simulink model "Encoder_Zynq_V25"  (R2021a)
settings: Solver=FixedStepDiscrete  StartTime=0.0  StopTime=SimulationsDauer  RelTol=1e-3
values from neighbouring files (symbols this model uses):
  f_ISR = 40e3    (= 40000)    [Script_Encoder_Zynq.m]
  IncPerTurn = 1024    [Script_Encoder_Zynq.m]
  inital_zero_speed_timeout = speed_timeout_in_s*f_fpga    (= 10000)    [Script_Encoder_Zynq.m]
  n_max = 6000    [Script_Encoder_Zynq.m]
  OmegaPerOverSampl = 500*((2*pi)/60)    (= 52.3598775598)    [Script_Encoder_Zynq.m]
  Periode = abs(1/Striche_pro_Sekunde)    [Script_Encoder_Zynq.m]
  Phase_Delay_A = Periode/8    [Script_Encoder_Zynq.m]
  Phase_Delay_B = -Periode/8    [Script_Encoder_Zynq.m]
  PolePair = 1    [Script_Encoder_Zynq.m]
  QuadratureFactor = 4    [Script_Encoder_Zynq.m]
  reciprocal_iterations = 3    [Script_Encoder_Zynq.m]
  T_50MHz = 1/f_50MHz    (= 1e-08)    [Script_Encoder_Zynq.m]
  T_mech = 1e-08    [Script_Encoder_Zynq.m]
undefined symbols (not defined in the file or in its folder): DiscIntNeverNeededParam, Newton, Raphson
libraries: hdlsllib x17, dspsrcs4 x3, simulink x2, dspswit3 x2, spsEdgeDetectorLib x2, simulink_extras x1, spspowerguiLib x1
(part 2 of 3)

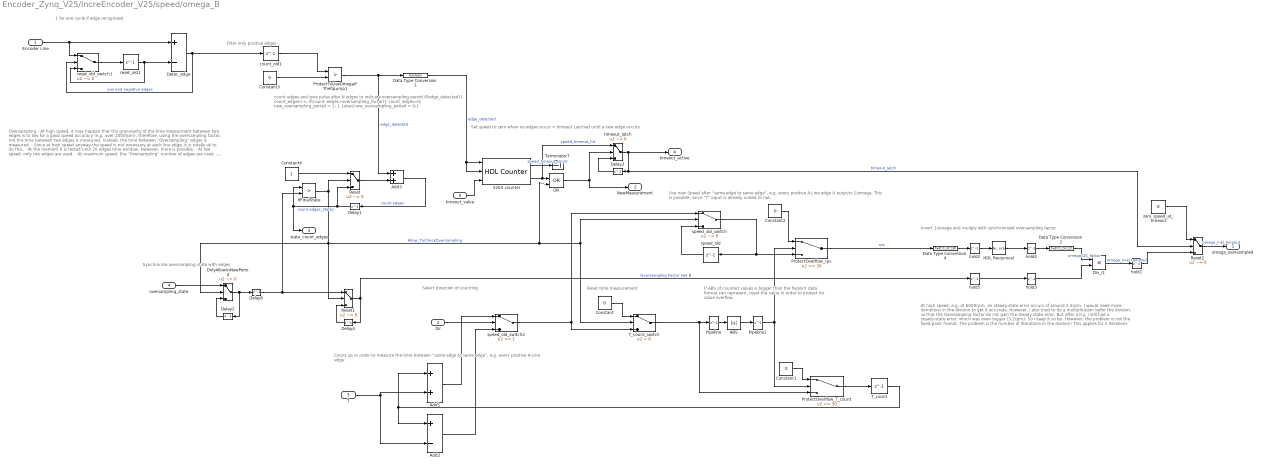
== system Encoder_Zynq_V25/IncreEncoder_V25/speed/omega_B ==
  note: Oversampling
      | - At high speed, it may happen that the granularity of the time measurment between
      | two edges is to low for a good speed accuracy (e.g. over 2000rpm), therefore, using
      | the oversampling factor, not the time between two edges is measured. Instead, the
      | time between "Oversampling" edges is measured.
      | - Since at high speed anyway the speed is not necessary at each line edge,
      |  it is totally ok to do this.
      | - At the moment it is tested until 20 edges time window. However, more is possible.
      | - At low speed, only two edges are used.
      | - At maximum speed, the "Oversampling" number of edges are used.
      | - Between them, a linear factor is used.
      | - Using the OverSampling number also at low speed is not possible,
      |  since the fixpoint range must be quite high! (fixdt(1,36,30) is used at the moment)
  note: Count up in order to measure the time between "same edge to same edge", e.g. every positive A-Line edge
  note: Reset time measurement
  note: 1 for one cycle if edge recognized
  note: Use new Speed after "same edge to same edge", e.g. every positive A-Line edge
      | It outputs 1/omega. This is possible, since "T" input is already scaled to rad.
  note: Select direction of counting
  note: If ABS of counted values is bigger than the
      | fixpoint data format can represent, reset the
      | value in order to protect for value overflow.
  note: Filter only positive edges
  note: count edges and give pulse after N edges to indicate oversampling period
      | if(edge_detected){
      | 	count_edges++;
      | 	if(count_edges>oversampling_factor){
      | 		count_edges=0;
      | 		new_oversampling_period = 1;
      | 	}
      | }else{new_oversampling_period = 0;}
  note: Synchronize oversampling state with edges
  note: At high speed, e.g. at 6000rpm, an steady-state error occurs of around 2.5rpm. I would need more iterrations in the division to get it accurate.
      | However, i also tried to do a multiplication befor the division, so that the Oversampling factor do not gain the steady-state error.
      | But after a try, i still had a steady-state error, which was even bigger (3,2rpm). So i keep it so far.
      | However, the problem is not the fixed-point fromat. The problem is the number of itterations in the division!
      | This applies for 3 iterations
  note: Invert 1/omega and muliply with synchronized oversampling factor
  note: Set speed to zero when no edges occur = timeout
      | Latched until a new edge occurs
  Encoder Line : Inport
  Dir : Inport  Port=2
  T : Inport  Port=3
  oversampling_state : Inport  Port=4
  timeout_value : Inport  Port=5  OutDataTypeStr=uint32
  32bit counter : hdlsllib/Sources/HDL Counter  CountType=Count limited  CountInit=0  CountStep=1  CountMax=inital_zero_speed_timeout  CountFromType=Initial value  CountFrom=0  CountResetPort=on  CountLoadPort=on  CountEnbPort=off  CountDirPort=off  CountHitOutputPort=on  CountDataType=Unsigned  CountWordLen=32  CountFracLen=0  CountSampTime=1
  ABS : Abs
  Add1 : Sum  OutDataTypeStr=Inherit: Same as first input
  Add2 : Sum  Inputs=+-  OutDataTypeStr=Inherit: Same as first input
  Add3 : Sum  OutDataTypeStr=Inherit: Same as accumulator
  Constant : Constant  Value=0  OutDataTypeStr=fixdt(1,38,32)  SampleTime=-1
  Constant1 : Constant  Value=0  OutDataTypeStr=fixdt(1,38,32)  SampleTime=-1
  Constant2 : Constant  Value=0  OutDataTypeStr=fixdt(1,38,32)  SampleTime=-1
  Constant3 : Constant  Value=0  OutDataTypeStr=int8  SampleTime=-1
  Constant4 : Constant  OutDataTypeStr=int8  SampleTime=T_50MHz
  Data Type Conversion1 : DataTypeConversion  OutDataTypeStr=boolean
  Data Type Conversion2 : DataTypeConversion  OutDataTypeStr=fixdt(1,24,12)
  Data Type Conversion4 : DataTypeConversion  OutDataTypeStr=fixdt(1,32,18)
  Delay{1..4,8} (5 alike) : Delay  DelayLength=1  InitialCondition=0
  Detec_edge : Sum  Inputs=+-  AccumDataTypeStr=int8  OutDataTypeStr=int8
  Div_i1 : Product  Inputs=**  OutDataTypeStr=fixdt(1,24,11)  RndMeth=Simplest  SaturateOnIntegerOverflow=on
  HDL Reciprocal : Reciprocal  NumberOfIterations=reciprocal_iterations
  IfFinalState : RelationalOperator  Operator=>  OutDataTypeStr=boolean  RndMeth=Nearest
  OR : Logic  Operator=OR  IconShape=distinctive  AllPortsSameDT=off  OutDataTypeStr=boolean
  OnlyAllowInNewPeriod : Switch  Criteria=u2 ~= 0  Threshold=0.5  OutDataTypeStr=fixdt(0,16,0)
  Pipeline : Delay  DelayLength=1
  Pipeline1 : Delay  DelayLength=1
  ProtectOverflow_T_count : Switch  Threshold=30
  ProtectOverflow_rps : Switch  Threshold=30  OutDataTypeStr=fixdt(1,38,32)
  ProtectToUseOmegaIfThetaJump1 : RelationalOperator  Operator=>  OutDataTypeStr=fixdt(1,16)  RndMeth=Nearest
  Reset : Switch  Criteria=u2 ~= 0  Threshold=0.5  OutDataTypeStr=fixdt(1,24,11)
  Reset1 : Switch  Criteria=u2 ~= 0  Threshold=0.5  OutDataTypeStr=Inherit: Inherit via back propagation
  Reset2 : Switch  Criteria=u2 ~= 0  Threshold=0.5  OutDataTypeStr=Inherit: Inherit via back propagation
  T_count : Delay  DelayLength=1
  T_count_switch : Switch  Criteria=u2 > Threshold
  Terminator7 : Terminator
  count_old1 : Delay  DelayLength=1
  hold1 : Delay
  hold{2..5} (4 alike) : Delay  DelayLength=1
  reset_old1 : Delay  DelayLength=1
  reset_old_switch1 : Switch  Criteria=u2 ~= 0
  speed_old : Delay  DelayLength=1
  speed_old_switch : Switch  Criteria=u2 ~= 0  OutDataTypeStr=fixdt(1,38,32)
  speed_old_switch2 : Switch  Threshold=1
  timeout_latch : Switch  Criteria=u2 ~= 0  Threshold=0.5  OutDataTypeStr=Inherit: Inherit via back propagation
  zero_speed_at_timeout : Constant  Value=0  OutDataTypeStr=fixdt(1,24,12)  SampleTime=-1
  omega_oversampled : Outport  VectorParamsAs1DForOutWhenUnconnected=off
  NewMeasurement : Outport  Port=2  VectorParamsAs1DForOutWhenUnconnected=off
  state_count_edges : Outport  Port=3  VectorParamsAs1DForOutWhenUnconnected=off
  timeout_active : Outport  Port=4  OutDataTypeStr=boolean  VectorParamsAs1DForOutWhenUnconnected=off
  wires:
  Constant/1 -> T_count_switch/1
  Constant1/1 -> ProtectOverflow_T_count/1
  Constant2/1 -> ProtectOverflow_rps/1
  speed_old_switch/1 -> ProtectOverflow_rps/3, speed_old/1
  speed_old/1 -> speed_old_switch/3
  T/1 -> Add1/2, Add2/2
  ProtectOverflow_T_count/1 -> T_count/1
  T_count/1 -> Add2/1, Add1/1
  speed_old_switch2/1 -> speed_old_switch/1, T_count_switch/3
  count_old1/1 -> ProtectToUseOmegaIfThetaJump1/1
  Constant3/1 -> ProtectToUseOmegaIfThetaJump1/2
  Encoder Line/1 -> reset_old_switch1/1, Detec_edge/1
  reset_old_switch1/1 -> reset_old1/1
  reset_old1/1 -> reset_old_switch1/3, Detec_edge/2
  Detec_edge/1 -> reset_old_switch1/2, count_old1/1  "pos and negative edges"
  Dir/1 -> speed_old_switch2/2
  Add1/1 -> speed_old_switch2/1
  Add2/1 -> speed_old_switch2/3
  T_count_switch/1 -> Pipeline/1, ProtectOverflow_T_count/3
  ABS/1 -> Pipeline1/1
  Pipeline/1 -> ABS/1
  Pipeline1/1 -> ProtectOverflow_T_count/2, ProtectOverflow_rps/2
  IfFinalState/1 -> OR/2, speed_old_switch/2, T_count_switch/2, Reset1/2, OnlyAllowInNewPeriod/2, Reset/2  "Allow_ToCheckOversampling"
  OnlyAllowInNewPeriod/1 -> Delay2/1, Delay8/1
  Delay1/1 -> Reset/3, state_count_edges/1, IfFinalState/1  "count edges_states"
  Add3/1 -> Delay1/1  "count edges"
  Reset/1 -> Add3/2
  Constant4/1 -> Reset/1
  Reset1/1 -> Delay4/1, hold5/1  "Oversampling Factor Not B"
  Delay2/1 -> OnlyAllowInNewPeriod/3
  oversampling_state/1 -> OnlyAllowInNewPeriod/1
  Delay4/1 -> Reset1/3
  Delay8/1 -> Reset1/1, IfFinalState/2
  ProtectToUseOmegaIfThetaJump1/1 -> Add3/1, Data Type Conversion1/1  "edge_detected"
  32bit counter/2 -> OR/1, timeout_latch/1  "speed_timeout_hit"
  OR/1 -> NewMeasurement/1, timeout_latch/2
  Div_i1/1 -> hold1/1  "omega_oversampled"
  hold2/1 -> HDL Reciprocal/1
  hold4/1 -> Data Type Conversion2/1
  HDL Reciprocal/1 -> hold4/1
  hold5/1 -> hold3/1
  hold3/1 -> Div_i1/2
  Data Type Conversion2/1 -> Div_i1/1  "omega/OS_factor"
  ProtectOverflow_rps/1 -> Data Type Conversion4/1  "rps"
  Data Type Conversion4/1 -> hold2/1
  zero_speed_at_timeout/1 -> Reset2/1
  Reset2/1 -> omega_oversampled/1  "omega_inkl_timeout"
  timeout_latch/1 -> timeout_active/1, Reset2/2, Delay3/1  "timeout_latch"
  Delay3/1 -> timeout_latch/3
  Data Type Conversion1/1 -> 32bit counter/2, 32bit counter/1  "edge_detected"
  timeout_value/1 -> 32bit counter/3
  32bit counter/1 -> Terminator7/1  "speed_timeout_count"
  hold1/1 -> Reset2/3

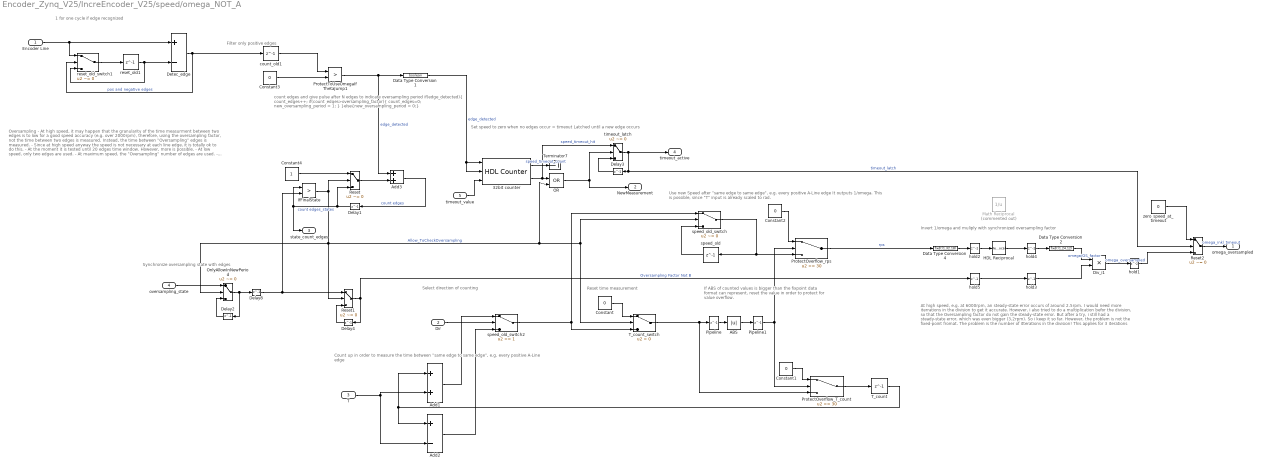
== system Encoder_Zynq_V25/IncreEncoder_V25/speed/omega_NOT_A ==
  note: Oversampling
      | - At high speed, it may happen that the granularity of the time measurment between
      | two edges is to low for a good speed accuracy (e.g. over 2000rpm), therefore, using
      | the oversampling factor, not the time between two edges is measured. Instead, the
      | time between "Oversampling" edges is measured.
      | - Since at high speed anyway the speed is not necessary at each line edge,
      |  it is totally ok to do this.
      | - At the moment it is tested until 20 edges time window. However, more is possible.
      | - At low speed, only two edges are used.
      | - At maximum speed, the "Oversampling" number of edges are used.
      | - Between them, a linear factor is used.
      | - Using the OverSampling number also at low speed is not possible,
      |  since the fixpoint range must be quite high! (fixdt(1,36,30) is used at the moment)
  note: Count up in order to measure the time between "same edge to same edge", e.g. every positive A-Line edge
  note: Reset time measurement
  note: 1 for one cycle if edge recognized
  note: Use new Speed after "same edge to same edge", e.g. every positive A-Line edge
      | It outputs 1/omega. This is possible, since "T" input is already scaled to rad.
  note: Select direction of counting
  note: If ABS of counted values is bigger than the
      | fixpoint data format can represent, reset the
      | value in order to protect for value overflow.
  note: Filter only positive edges
  note: count edges and give pulse after N edges to indicate oversampling period
      | if(edge_detected){
      | 	count_edges++;
      | 	if(count_edges>oversampling_factor){
      | 		count_edges=0;
      | 		new_oversampling_period = 1;
      | 	}
      | }else{new_oversampling_period = 0;}
  note: Synchronize oversampling state with edges
  note: At high speed, e.g. at 6000rpm, an steady-state error occurs of around 2.5rpm. I would need more iterrations in the division to get it accurate.
      | However, i also tried to do a multiplication befor the division, so that the Oversampling factor do not gain the steady-state error.
      | But after a try, i still had a steady-state error, which was even bigger (3,2rpm). So i keep it so far.
      | However, the problem is not the fixed-point fromat. The problem is the number of itterations in the division!
      | This applies for 3 iterations
  note: Invert 1/omega and muliply with synchronized oversampling factor
  note: Set speed to zero when no edges occur = timeout
      | Latched until a new edge occurs
  Encoder Line : Inport
  Dir : Inport  Port=2
  T : Inport  Port=3
  oversampling_state : Inport  Port=4
  timeout_value : Inport  Port=5  OutDataTypeStr=uint32
  32bit counter : hdlsllib/Sources/HDL Counter  CountType=Count limited  CountInit=0  CountStep=1  CountMax=inital_zero_speed_timeout  CountFromType=Initial value  CountFrom=0  CountResetPort=on  CountLoadPort=on  CountEnbPort=off  CountDirPort=off  CountHitOutputPort=on  CountDataType=Unsigned  CountWordLen=32  CountFracLen=0  CountSampTime=1
  ABS : Abs
  Add1 : Sum  OutDataTypeStr=Inherit: Same as first input
  Add2 : Sum  Inputs=+-  OutDataTypeStr=Inherit: Same as first input
  Add3 : Sum  OutDataTypeStr=Inherit: Same as accumulator
  Constant : Constant  Value=0  OutDataTypeStr=fixdt(1,38,32)  SampleTime=-1
  Constant1 : Constant  Value=0  OutDataTypeStr=fixdt(1,38,32)  SampleTime=-1
  Constant2 : Constant  Value=0  OutDataTypeStr=fixdt(1,38,32)  SampleTime=-1
  Constant3 : Constant  Value=0  OutDataTypeStr=int8  SampleTime=-1
  Constant4 : Constant  OutDataTypeStr=int8  SampleTime=T_50MHz
  Data Type Conversion1 : DataTypeConversion  OutDataTypeStr=boolean
  Data Type Conversion2 : DataTypeConversion  OutDataTypeStr=fixdt(1,24,12)
  Data Type Conversion4 : DataTypeConversion  OutDataTypeStr=fixdt(1,32,18)
  Delay{1..4,8} (5 alike) : Delay  DelayLength=1  InitialCondition=0
  Detec_edge : Sum  Inputs=+-  AccumDataTypeStr=int8  OutDataTypeStr=int8
  Div_i1 : Product  Inputs=**  OutDataTypeStr=fixdt(1,24,11)  RndMeth=Simplest  SaturateOnIntegerOverflow=on
  HDL Reciprocal : Reciprocal  NumberOfIterations=reciprocal_iterations
  IfFinalState : RelationalOperator  Operator=>  OutDataTypeStr=boolean  RndMeth=Nearest
  Math Reciprocal : Math  Commented=on  Operator=reciprocal  AlgorithmMethod=Newton-Raphson  SignedPower=on  Iterations=reciprocal_iterations  SaturateOnIntegerOverflow=on
  OR : Logic  Operator=OR  IconShape=distinctive  AllPortsSameDT=off  OutDataTypeStr=boolean
  OnlyAllowInNewPeriod : Switch  Criteria=u2 ~= 0  Threshold=0.5  OutDataTypeStr=fixdt(0,16,0)
  Pipeline : Delay  DelayLength=1
  Pipeline1 : Delay  DelayLength=1
  ProtectOverflow_T_count : Switch  Threshold=30
  ProtectOverflow_rps : Switch  Threshold=30  OutDataTypeStr=fixdt(1,38,32)
  ProtectToUseOmegaIfThetaJump1 : RelationalOperator  Operator=>  OutDataTypeStr=fixdt(1,16)  RndMeth=Nearest
  Reset : Switch  Criteria=u2 ~= 0  Threshold=0.5  OutDataTypeStr=fixdt(1,24,11)
  Reset1 : Switch  Criteria=u2 ~= 0  Threshold=0.5  OutDataTypeStr=Inherit: Inherit via back propagation
  Reset2 : Switch  Criteria=u2 ~= 0  Threshold=0.5  OutDataTypeStr=Inherit: Inherit via back propagation
  T_count : Delay  DelayLength=1
  T_count_switch : Switch  Criteria=u2 > Threshold
  Terminator7 : Terminator
  count_old1 : Delay  DelayLength=1
  hold1 : Delay
  hold{2..5} (4 alike) : Delay  DelayLength=1
  reset_old1 : Delay  DelayLength=1
  reset_old_switch1 : Switch  Criteria=u2 ~= 0
  speed_old : Delay  DelayLength=1
  speed_old_switch : Switch  Criteria=u2 ~= 0  OutDataTypeStr=fixdt(1,38,32)
  speed_old_switch2 : Switch  Threshold=1
  timeout_latch : Switch  Criteria=u2 ~= 0  Threshold=0.5  OutDataTypeStr=Inherit: Inherit via back propagation
  zero_speed_at_timeout : Constant  Value=0  OutDataTypeStr=fixdt(1,24,12)  SampleTime=-1
  omega_oversampled : Outport  VectorParamsAs1DForOutWhenUnconnected=off
  NewMeasurement : Outport  Port=2  VectorParamsAs1DForOutWhenUnconnected=off
  state_count_edges : Outport  Port=3  VectorParamsAs1DForOutWhenUnconnected=off
  timeout_active : Outport  Port=4  OutDataTypeStr=boolean  VectorParamsAs1DForOutWhenUnconnected=off
  wires:
  Constant/1 -> T_count_switch/1
  Constant1/1 -> ProtectOverflow_T_count/1
  Constant2/1 -> ProtectOverflow_rps/1
  speed_old_switch/1 -> ProtectOverflow_rps/3, speed_old/1
  speed_old/1 -> speed_old_switch/3
  T/1 -> Add1/2, Add2/2
  ProtectOverflow_T_count/1 -> T_count/1
  T_count/1 -> Add2/1, Add1/1
  speed_old_switch2/1 -> speed_old_switch/1, T_count_switch/3
  count_old1/1 -> ProtectToUseOmegaIfThetaJump1/1
  Constant3/1 -> ProtectToUseOmegaIfThetaJump1/2
  Encoder Line/1 -> reset_old_switch1/1, Detec_edge/1
  reset_old_switch1/1 -> reset_old1/1
  reset_old1/1 -> reset_old_switch1/3, Detec_edge/2
  Detec_edge/1 -> reset_old_switch1/2, count_old1/1  "pos and negative edges"
  Dir/1 -> speed_old_switch2/2
  Add1/1 -> speed_old_switch2/1
  Add2/1 -> speed_old_switch2/3
  T_count_switch/1 -> Pipeline/1, ProtectOverflow_T_count/3
  ABS/1 -> Pipeline1/1
  Pipeline/1 -> ABS/1
  Pipeline1/1 -> ProtectOverflow_T_count/2, ProtectOverflow_rps/2
  IfFinalState/1 -> OR/2, speed_old_switch/2, T_count_switch/2, Reset1/2, OnlyAllowInNewPeriod/2, Reset/2  "Allow_ToCheckOversampling"
  OnlyAllowInNewPeriod/1 -> Delay2/1, Delay8/1
  Delay1/1 -> Reset/3, state_count_edges/1, IfFinalState/1  "count edges_states"
  Add3/1 -> Delay1/1  "count edges"
  Reset/1 -> Add3/2
  Constant4/1 -> Reset/1
  Reset1/1 -> Delay4/1, hold5/1  "Oversampling Factor Not B"
  Delay2/1 -> OnlyAllowInNewPeriod/3
  oversampling_state/1 -> OnlyAllowInNewPeriod/1
  Delay4/1 -> Reset1/3
  Delay8/1 -> Reset1/1, IfFinalState/2
  ProtectToUseOmegaIfThetaJump1/1 -> Add3/1, Data Type Conversion1/1  "edge_detected"
  32bit counter/2 -> OR/1, timeout_latch/1  "speed_timeout_hit"
  OR/1 -> NewMeasurement/1, timeout_latch/2
  Div_i1/1 -> hold1/1  "omega_oversampled"
  hold2/1 -> HDL Reciprocal/1
  hold4/1 -> Data Type Conversion2/1
  HDL Reciprocal/1 -> hold4/1
  hold5/1 -> hold3/1
  hold3/1 -> Div_i1/2
  Data Type Conversion2/1 -> Div_i1/1  "omega/OS_factor"
  ProtectOverflow_rps/1 -> Data Type Conversion4/1  "rps"
  Data Type Conversion4/1 -> hold2/1
  zero_speed_at_timeout/1 -> Reset2/1
  Reset2/1 -> omega_oversampled/1  "omega_inkl_timeout"
  timeout_latch/1 -> timeout_active/1, Reset2/2, Delay3/1  "timeout_latch"
  Delay3/1 -> timeout_latch/3
  Data Type Conversion1/1 -> 32bit counter/2, 32bit counter/1  "edge_detected"
  timeout_value/1 -> 32bit counter/3
  32bit counter/1 -> Terminator7/1  "speed_timeout_count"
  hold1/1 -> Reset2/3

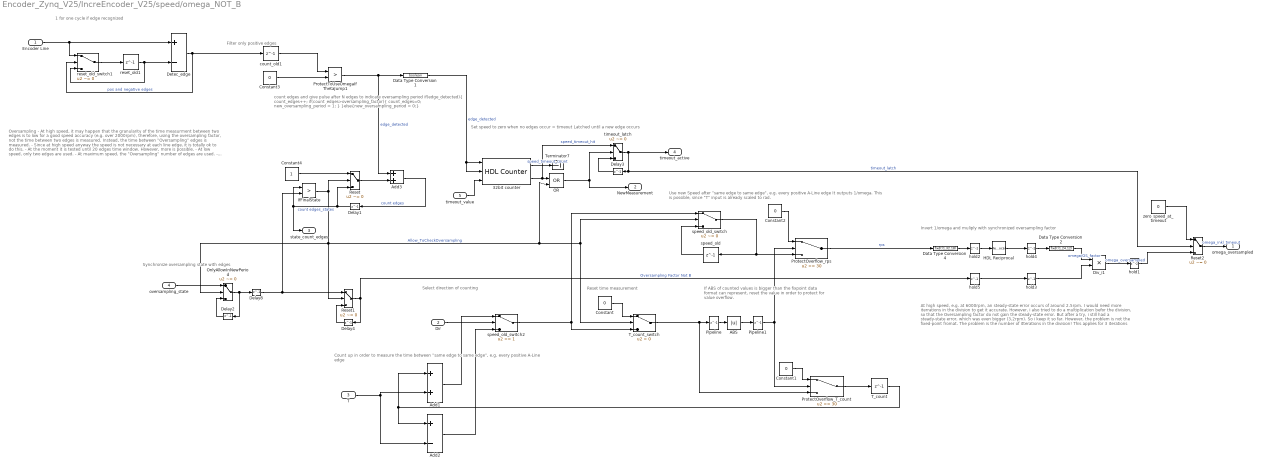
== system Encoder_Zynq_V25/IncreEncoder_V25/speed/omega_NOT_B ==
  note: Oversampling
      | - At high speed, it may happen that the granularity of the time measurment between
      | two edges is to low for a good speed accuracy (e.g. over 2000rpm), therefore, using
      | the oversampling factor, not the time between two edges is measured. Instead, the
      | time between "Oversampling" edges is measured.
      | - Since at high speed anyway the speed is not necessary at each line edge,
      |  it is totally ok to do this.
      | - At the moment it is tested until 20 edges time window. However, more is possible.
      | - At low speed, only two edges are used.
      | - At maximum speed, the "Oversampling" number of edges are used.
      | - Between them, a linear factor is used.
      | - Using the OverSampling number also at low speed is not possible,
      |  since the fixpoint range must be quite high! (fixdt(1,36,30) is used at the moment)
  note: Count up in order to measure the time between "same edge to same edge", e.g. every positive A-Line edge
  note: Reset time measurement
  note: 1 for one cycle if edge recognized
  note: Use new Speed after "same edge to same edge", e.g. every positive A-Line edge
      | It outputs 1/omega. This is possible, since "T" input is already scaled to rad.
  note: Select direction of counting
  note: If ABS of counted values is bigger than the
      | fixpoint data format can represent, reset the
      | value in order to protect for value overflow.
  note: Filter only positive edges
  note: count edges and give pulse after N edges to indicate oversampling period
      | if(edge_detected){
      | 	count_edges++;
      | 	if(count_edges>oversampling_factor){
      | 		count_edges=0;
      | 		new_oversampling_period = 1;
      | 	}
      | }else{new_oversampling_period = 0;}
  note: Synchronize oversampling state with edges
  note: At high speed, e.g. at 6000rpm, an steady-state error occurs of around 2.5rpm. I would need more iterrations in the division to get it accurate.
      | However, i also tried to do a multiplication befor the division, so that the Oversampling factor do not gain the steady-state error.
      | But after a try, i still had a steady-state error, which was even bigger (3,2rpm). So i keep it so far.
      | However, the problem is not the fixed-point fromat. The problem is the number of itterations in the division!
      | This applies for 3 iterations
  note: Invert 1/omega and muliply with synchronized oversampling factor
  note: Set speed to zero when no edges occur = timeout
      | Latched until a new edge occurs
  Encoder Line : Inport
  Dir : Inport  Port=2
  T : Inport  Port=3
  oversampling_state : Inport  Port=4
  timeout_value : Inport  Port=5  OutDataTypeStr=uint32
  32bit counter : hdlsllib/Sources/HDL Counter  CountType=Count limited  CountInit=0  CountStep=1  CountMax=inital_zero_speed_timeout  CountFromType=Initial value  CountFrom=0  CountResetPort=on  CountLoadPort=on  CountEnbPort=off  CountDirPort=off  CountHitOutputPort=on  CountDataType=Unsigned  CountWordLen=32  CountFracLen=0  CountSampTime=1
  ABS : Abs
  Add1 : Sum  OutDataTypeStr=Inherit: Same as first input
  Add2 : Sum  Inputs=+-  OutDataTypeStr=Inherit: Same as first input
  Add3 : Sum  OutDataTypeStr=Inherit: Same as accumulator
  Constant : Constant  Value=0  OutDataTypeStr=fixdt(1,38,32)  SampleTime=-1
  Constant1 : Constant  Value=0  OutDataTypeStr=fixdt(1,38,32)  SampleTime=-1
  Constant2 : Constant  Value=0  OutDataTypeStr=fixdt(1,38,32)  SampleTime=-1
  Constant3 : Constant  Value=0  OutDataTypeStr=int8  SampleTime=-1
  Constant4 : Constant  OutDataTypeStr=int8  SampleTime=T_50MHz
  Data Type Conversion1 : DataTypeConversion  OutDataTypeStr=boolean
  Data Type Conversion2 : DataTypeConversion  OutDataTypeStr=fixdt(1,24,12)
  Data Type Conversion4 : DataTypeConversion  OutDataTypeStr=fixdt(1,32,18)
  Delay{1..4,8} (5 alike) : Delay  DelayLength=1  InitialCondition=0
  Detec_edge : Sum  Inputs=+-  AccumDataTypeStr=int8  OutDataTypeStr=int8
  Div_i1 : Product  Inputs=**  OutDataTypeStr=fixdt(1,24,11)  RndMeth=Simplest  SaturateOnIntegerOverflow=on
  HDL Reciprocal : Reciprocal  NumberOfIterations=reciprocal_iterations
  IfFinalState : RelationalOperator  Operator=>  OutDataTypeStr=boolean  RndMeth=Nearest
  OR : Logic  Operator=OR  IconShape=distinctive  AllPortsSameDT=off  OutDataTypeStr=boolean
  OnlyAllowInNewPeriod : Switch  Criteria=u2 ~= 0  Threshold=0.5  OutDataTypeStr=fixdt(0,16,0)
  Pipeline : Delay  DelayLength=1
  Pipeline1 : Delay  DelayLength=1
  ProtectOverflow_T_count : Switch  Threshold=30
  ProtectOverflow_rps : Switch  Threshold=30  OutDataTypeStr=fixdt(1,38,32)
  ProtectToUseOmegaIfThetaJump1 : RelationalOperator  Operator=>  OutDataTypeStr=fixdt(1,16)  RndMeth=Nearest
  Reset : Switch  Criteria=u2 ~= 0  Threshold=0.5  OutDataTypeStr=fixdt(1,24,11)
  Reset1 : Switch  Criteria=u2 ~= 0  Threshold=0.5  OutDataTypeStr=Inherit: Inherit via back propagation
  Reset2 : Switch  Criteria=u2 ~= 0  Threshold=0.5  OutDataTypeStr=Inherit: Inherit via back propagation
  T_count : Delay  DelayLength=1
  T_count_switch : Switch  Criteria=u2 > Threshold
  Terminator7 : Terminator
  count_old1 : Delay  DelayLength=1
  hold1 : Delay
  hold{2..5} (4 alike) : Delay  DelayLength=1
  reset_old1 : Delay  DelayLength=1
  reset_old_switch1 : Switch  Criteria=u2 ~= 0
  speed_old : Delay  DelayLength=1
  speed_old_switch : Switch  Criteria=u2 ~= 0  OutDataTypeStr=fixdt(1,38,32)
  speed_old_switch2 : Switch  Threshold=1
  timeout_latch : Switch  Criteria=u2 ~= 0  Threshold=0.5  OutDataTypeStr=Inherit: Inherit via back propagation
  zero_speed_at_timeout : Constant  Value=0  OutDataTypeStr=fixdt(1,24,12)  SampleTime=-1
  omega_oversampled : Outport  VectorParamsAs1DForOutWhenUnconnected=off
  NewMeasurement : Outport  Port=2  VectorParamsAs1DForOutWhenUnconnected=off
  state_count_edges : Outport  Port=3  VectorParamsAs1DForOutWhenUnconnected=off
  timeout_active : Outport  Port=4  OutDataTypeStr=boolean  VectorParamsAs1DForOutWhenUnconnected=off
  wires:
  Constant/1 -> T_count_switch/1
  Constant1/1 -> ProtectOverflow_T_count/1
  Constant2/1 -> ProtectOverflow_rps/1
  speed_old_switch/1 -> ProtectOverflow_rps/3, speed_old/1
  speed_old/1 -> speed_old_switch/3
  T/1 -> Add1/2, Add2/2
  ProtectOverflow_T_count/1 -> T_count/1
  T_count/1 -> Add2/1, Add1/1
  speed_old_switch2/1 -> speed_old_switch/1, T_count_switch/3
  count_old1/1 -> ProtectToUseOmegaIfThetaJump1/1
  Constant3/1 -> ProtectToUseOmegaIfThetaJump1/2
  Encoder Line/1 -> reset_old_switch1/1, Detec_edge/1
  reset_old_switch1/1 -> reset_old1/1
  reset_old1/1 -> reset_old_switch1/3, Detec_edge/2
  Detec_edge/1 -> reset_old_switch1/2, count_old1/1  "pos and negative edges"
  Dir/1 -> speed_old_switch2/2
  Add1/1 -> speed_old_switch2/1
  Add2/1 -> speed_old_switch2/3
  T_count_switch/1 -> Pipeline/1, ProtectOverflow_T_count/3
  ABS/1 -> Pipeline1/1
  Pipeline/1 -> ABS/1
  Pipeline1/1 -> ProtectOverflow_T_count/2, ProtectOverflow_rps/2
  IfFinalState/1 -> OR/2, speed_old_switch/2, T_count_switch/2, Reset1/2, OnlyAllowInNewPeriod/2, Reset/2  "Allow_ToCheckOversampling"
  OnlyAllowInNewPeriod/1 -> Delay2/1, Delay8/1
  Delay1/1 -> Reset/3, state_count_edges/1, IfFinalState/1  "count edges_states"
  Add3/1 -> Delay1/1  "count edges"
  Reset/1 -> Add3/2
  Constant4/1 -> Reset/1
  Reset1/1 -> Delay4/1, hold5/1  "Oversampling Factor Not B"
  Delay2/1 -> OnlyAllowInNewPeriod/3
  oversampling_state/1 -> OnlyAllowInNewPeriod/1
  Delay4/1 -> Reset1/3
  Delay8/1 -> Reset1/1, IfFinalState/2
  ProtectToUseOmegaIfThetaJump1/1 -> Add3/1, Data Type Conversion1/1  "edge_detected"
  32bit counter/2 -> OR/1, timeout_latch/1  "speed_timeout_hit"
  OR/1 -> NewMeasurement/1, timeout_latch/2
  Div_i1/1 -> hold1/1  "omega_oversampled"
  hold2/1 -> HDL Reciprocal/1
  hold4/1 -> Data Type Conversion2/1
  HDL Reciprocal/1 -> hold4/1
  hold5/1 -> hold3/1
  hold3/1 -> Div_i1/2
  Data Type Conversion2/1 -> Div_i1/1  "omega/OS_factor"
  ProtectOverflow_rps/1 -> Data Type Conversion4/1  "rps"
  Data Type Conversion4/1 -> hold2/1
  zero_speed_at_timeout/1 -> Reset2/1
  Reset2/1 -> omega_oversampled/1  "omega_inkl_timeout"
  timeout_latch/1 -> timeout_active/1, Reset2/2, Delay3/1  "timeout_latch"
  Delay3/1 -> timeout_latch/3
  Data Type Conversion1/1 -> 32bit counter/2, 32bit counter/1  "edge_detected"
  timeout_value/1 -> 32bit counter/3
  32bit counter/1 -> Terminator7/1  "speed_timeout_count"
  hold1/1 -> Reset2/3

== system Encoder_Zynq_V25/IncreEncoder_V25/speed/omega_by_time_oversampled_NOT_A22 ==
  note: At high speed, e.g. at 6000rpm, an steady-state error occurs of around 2.5rpm. I would need more iterrations in the division to get it accurate.
      | However, i also tried to do a multiplication befor the division, so that the Oversampling factor do not gain the steady-state error.
      | But after a try, i still had a steady-state error, which was even bigger (3,2rpm). So i keep it so far.
      | However, the problem is not the fixed-point fromat. The problem is the number of itterations in the division!
      | This applies for 3 iterations
  Encoder Line : Inport
  Dir : Inport  Port=2
  T : Inport  Port=3
  oversampling_state : Inport  Port=4
  Average_linear_Reg : Subsystem  Commented=on
  Data Type Conversion2 : DataTypeConversion  OutDataTypeStr=fixdt(1,24,12)
  Data Type Conversion4 : DataTypeConversion  OutDataTypeStr=fixdt(1,32,18)
  Div_i1 : Product  Inputs=**  OutDataTypeStr=fixdt(1,24,11)  RndMeth=Simplest  SaturateOnIntegerOverflow=on
  HDL Reciprocal : Reciprocal  NumberOfIterations=reciprocal_iterations
  hold{2..5} (4 alike) : Delay  DelayLength=1
  omega_by_measure_time : Subsystem  TreatAsAtomicUnit=on
  omega_oversampled1 : Outport
  New Measurement : Outport  Port=2
  state_count_edges : Outport  Port=3  VectorParamsAs1DForOutWhenUnconnected=off
  wires:
  Data Type Conversion4/1 -> hold2/1
  hold3/1 -> Div_i1/2
  omega_by_measure_time/1(one_Omega) -> Data Type Conversion4/1  "rps"
  hold2/1 -> HDL Reciprocal/1
  Div_i1/1 -> omega_oversampled1/1  "omega_oversampled"
  Data Type Conversion2/1 -> Div_i1/1  "omega_oversampled"
  hold4/1 -> Data Type Conversion2/1
  hold5/1 -> hold3/1
  Encoder Line/1 -> omega_by_measure_time/1(Encoder Line)
  omega_by_measure_time/2(OverSamplingFactor) -> hold5/1
  omega_by_measure_time/3(NewMeasurement) -> New Measurement/1  "NewMeasurement"
  HDL Reciprocal/1 -> hold4/1
  Dir/1 -> omega_by_measure_time/3(Dir)
  T/1 -> omega_by_measure_time/2(T)
  oversampling_state/1 -> omega_by_measure_time/4(oversampling_state)
  omega_by_measure_time/4(state_count_edges) -> state_count_edges/1

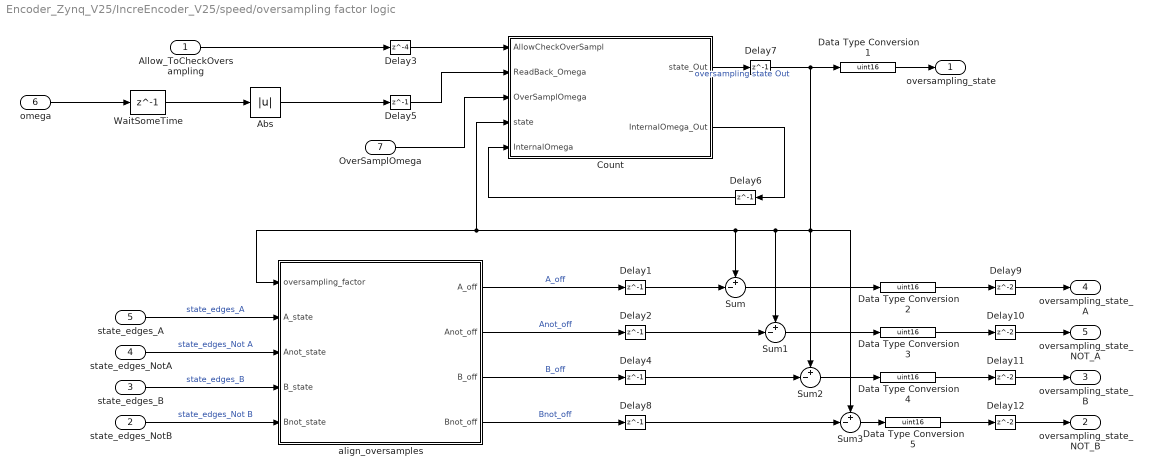
== system Encoder_Zynq_V25/IncreEncoder_V25/speed/oversampling factor logic ==
  Allow_ToCheckOversampling : Inport
  state_edges_NotB : Inport  Port=2
  state_edges_B : Inport  Port=3
  state_edges_NotA : Inport  Port=4
  state_edges_A : Inport  Port=5
  omega : Inport  Port=6
  OverSamplOmega : Inport  Port=7
  Abs : Abs
  Count : MATLAB Function  TreatAsAtomicUnit=on
  Data Type Conversion{1..5} (5 alike) : DataTypeConversion  OutDataTypeStr=uint16
  Delay{1..2,4,7..8} (5 alike) : Delay  DelayLength=1  InitialCondition=1
  Delay{9..12} (4 alike) : Delay  InitialCondition=1
  Delay3 : Delay  DelayLength=4  InitialCondition=0
  Delay5 : Delay  DelayLength=1  InitialCondition=0
  Delay6 : Delay  DelayLength=1  InitialCondition=0
  Sum{,1..3} (4 alike) : Sum  Inputs=+-|  AccumDataTypeStr=uint16
  WaitSomeTime : Delay  DelayLength=1
  align_oversamples : MATLAB Function  TreatAsAtomicUnit=on
  oversampling_state : Outport
  oversampling_state_NOT_B : Outport  Port=2
  oversampling_state_B : Outport  Port=3
  oversampling_state_A : Outport  Port=4
  oversampling_state_NOT_A : Outport  Port=5
  wires:
  OverSamplOmega/1 -> Count/3(OverSamplOmega)
  Count/1(state_Out) -> Delay7/1  "oversampling state Out"
  WaitSomeTime/1 -> Abs/1
  Count/2(InternalOmega_Out) -> Delay6/1
  Delay6/1 -> Count/5(InternalOmega)
  Abs/1 -> Delay5/1
  Delay5/1 -> Count/2(ReadBack_Omega)
  Delay3/1 -> Count/1(AllowCheckOverSampl)
  omega/1 -> WaitSomeTime/1
  Allow_ToCheckOversampling/1 -> Delay3/1
  Delay7/1 -> Sum1/1, align_oversamples/1(oversampling_factor), Count/4(state), Sum/1, Sum2/1, Sum3/1, Data Type Conversion1/1
  Data Type Conversion1/1 -> oversampling_state/1
  state_edges_A/1 -> align_oversamples/2(A_state)  "state_edges_A"
  state_edges_NotA/1 -> align_oversamples/3(Anot_state)  "state_edges_Not A"
  state_edges_B/1 -> align_oversamples/4(B_state)  "state_edges_B"
  state_edges_NotB/1 -> align_oversamples/5(Bnot_state)  "state_edges_Not B"
  Sum/1 -> Data Type Conversion2/1
  align_oversamples/1(A_off) -> Delay1/1  "A_off"
  align_oversamples/2(Anot_off) -> Delay2/1  "Anot_off"
  align_oversamples/3(B_off) -> Delay4/1  "B_off"
  align_oversamples/4(Bnot_off) -> Delay8/1  "Bnot_off"
  Sum3/1 -> Data Type Conversion5/1
  Sum2/1 -> Data Type Conversion4/1
  Sum1/1 -> Data Type Conversion3/1
  Data Type Conversion2/1 -> Delay9/1
  Delay1/1 -> Sum/2
  Delay2/1 -> Sum1/2
  Delay4/1 -> Sum2/2
  Delay8/1 -> Sum3/2
  Data Type Conversion5/1 -> Delay12/1
  Delay12/1 -> oversampling_state_NOT_B/1
  Data Type Conversion4/1 -> Delay11/1
  Delay11/1 -> oversampling_state_B/1
  Delay10/1 -> oversampling_state_NOT_A/1
  Data Type Conversion3/1 -> Delay10/1
  Delay9/1 -> oversampling_state_A/1

== system Encoder_Zynq_V25/IncrementalEncoder_Floating/n_aus_theta_v4/Geschwindigkeitsfilter1 ==
  In1 : Inport
  Add1 : Sum  Inputs=+-
  Discrete-Time Integrator2 : DiscreteIntegrator  SampleTime=-1  ICPrevOutput=DiscIntNeverNeededParam  ICPrevScaledInput=DiscIntNeverNeededParam
  Gain2 2500 10000 : Gain  Gain=10000
  Scope1 : Scope  NumInputPorts=5
  Out1 : Outport  InitialOutput=[0]  VectorParamsAs1DForOutWhenUnconnected=off
  wires:
  Add1/1 -> Scope1/4, Gain2 2500 10000/1
  Gain2 2500 10000/1 -> Scope1/3, Discrete-Time Integrator2/1
  Discrete-Time Integrator2/1 -> Scope1/2, Out1/1, Add1/2
  In1/1 -> Scope1/5, Add1/1

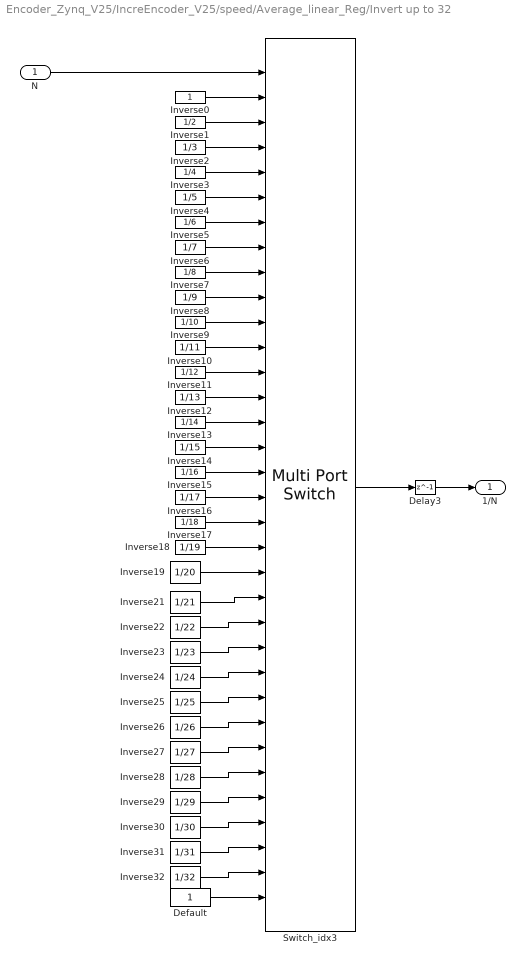
== system Encoder_Zynq_V25/IncreEncoder_V25/speed/Average_linear_Reg/Invert up to 32 ==
  N : Inport
  Default : Constant  OutDataTypeStr=fixdt(0,18,18)  SampleTime=-1
  Delay3 : Delay  DelayLength=1  InitialCondition=0
  Inverse0 : Constant  OutDataTypeStr=fixdt(0,18,18)  SampleTime=-1
  Inverse1 : Constant  Value=1/2  OutDataTypeStr=fixdt(0,18,18)  SampleTime=-1
  Inverse10 : Constant  Value=1/11  OutDataTypeStr=fixdt(0,18,18)  SampleTime=-1
  Inverse11 : Constant  Value=1/12  OutDataTypeStr=fixdt(0,18,18)  SampleTime=-1
  Inverse12 : Constant  Value=1/13  OutDataTypeStr=fixdt(0,18,18)  SampleTime=-1
  Inverse13 : Constant  Value=1/14  OutDataTypeStr=fixdt(0,18,18)  SampleTime=-1
  Inverse14 : Constant  Value=1/15  OutDataTypeStr=fixdt(0,18,18)  SampleTime=-1
  Inverse15 : Constant  Value=1/16  OutDataTypeStr=fixdt(0,18,18)  SampleTime=-1
  Inverse16 : Constant  Value=1/17  OutDataTypeStr=fixdt(0,18,18)  SampleTime=-1
  Inverse17 : Constant  Value=1/18  OutDataTypeStr=fixdt(0,18,18)  SampleTime=-1
  Inverse18 : Constant  Value=1/19  OutDataTypeStr=fixdt(0,18,18)  SampleTime=-1
  Inverse19 : Constant  Value=1/20  OutDataTypeStr=fixdt(0,18,18)  SampleTime=-1
  Inverse2 : Constant  Value=1/3  OutDataTypeStr=fixdt(0,18,18)  SampleTime=-1
  Inverse21 : Constant  Value=1/21  OutDataTypeStr=fixdt(0,18,18)  SampleTime=-1
  Inverse22 : Constant  Value=1/22  OutDataTypeStr=fixdt(0,18,18)  SampleTime=-1
  Inverse23 : Constant  Value=1/23  OutDataTypeStr=fixdt(0,18,18)  SampleTime=-1
  Inverse24 : Constant  Value=1/24  OutDataTypeStr=fixdt(0,18,18)  SampleTime=-1
  Inverse25 : Constant  Value=1/25  OutDataTypeStr=fixdt(0,18,18)  SampleTime=-1
  Inverse26 : Constant  Value=1/26  OutDataTypeStr=fixdt(0,18,18)  SampleTime=-1
  Inverse27 : Constant  Value=1/27  OutDataTypeStr=fixdt(0,18,18)  SampleTime=-1
  Inverse28 : Constant  Value=1/28  OutDataTypeStr=fixdt(0,18,18)  SampleTime=-1
  Inverse29 : Constant  Value=1/29  OutDataTypeStr=fixdt(0,18,18)  SampleTime=-1
  Inverse3 : Constant  Value=1/4  OutDataTypeStr=fixdt(0,18,18)  SampleTime=-1
  Inverse30 : Constant  Value=1/30  OutDataTypeStr=fixdt(0,18,18)  SampleTime=-1
  Inverse31 : Constant  Value=1/31  OutDataTypeStr=fixdt(0,18,18)  SampleTime=-1
  Inverse32 : Constant  Value=1/32  OutDataTypeStr=fixdt(0,18,18)  SampleTime=-1
  Inverse4 : Constant  Value=1/5  OutDataTypeStr=fixdt(0,18,18)  SampleTime=-1
  Inverse5 : Constant  Value=1/6  OutDataTypeStr=fixdt(0,18,18)  SampleTime=-1
  Inverse6 : Constant  Value=1/7  OutDataTypeStr=fixdt(0,18,18)  SampleTime=-1
  Inverse7 : Constant  Value=1/8  OutDataTypeStr=fixdt(0,18,18)  SampleTime=-1
  Inverse8 : Constant  Value=1/9  OutDataTypeStr=fixdt(0,18,18)  SampleTime=-1
  Inverse9 : Constant  Value=1/10  OutDataTypeStr=fixdt(0,18,18)  SampleTime=-1
  Switch_idx3 : MultiPortSwitch  Inputs=32  DataPortForDefault=Additional data port  DiagnosticForDefault=None  OutDataTypeStr=fixdt(0,18,18)  RndMeth=Simplest
  1/N : Outport
  wires:
  Inverse31/1 -> Switch_idx3/32
  Inverse3/1 -> Switch_idx3/5
  Inverse27/1 -> Switch_idx3/28
  Inverse1/1 -> Switch_idx3/3
  N/1 -> Switch_idx3/1
  Inverse14/1 -> Switch_idx3/16
  Inverse12/1 -> Switch_idx3/14
  Inverse19/1 -> Switch_idx3/21
  Inverse13/1 -> Switch_idx3/15
  Inverse6/1 -> Switch_idx3/8
  Inverse16/1 -> Switch_idx3/18
  Inverse4/1 -> Switch_idx3/6
  Inverse17/1 -> Switch_idx3/19
  Switch_idx3/1 -> Delay3/1
  Inverse15/1 -> Switch_idx3/17
  Inverse28/1 -> Switch_idx3/29
  Inverse2/1 -> Switch_idx3/4
  Inverse5/1 -> Switch_idx3/7
  Inverse8/1 -> Switch_idx3/10
  Inverse11/1 -> Switch_idx3/13
  Inverse9/1 -> Switch_idx3/11
  Inverse7/1 -> Switch_idx3/9
  Inverse10/1 -> Switch_idx3/12
  Inverse25/1 -> Switch_idx3/26
  Default/1 -> Switch_idx3/34
  Inverse21/1 -> Switch_idx3/22
  Inverse24/1 -> Switch_idx3/25
  Inverse26/1 -> Switch_idx3/27
  Inverse18/1 -> Switch_idx3/20
  Inverse0/1 -> Switch_idx3/2
  Inverse29/1 -> Switch_idx3/30
  Inverse22/1 -> Switch_idx3/23
  Inverse32/1 -> Switch_idx3/33
  Inverse30/1 -> Switch_idx3/31
  Inverse23/1 -> Switch_idx3/24
  Delay3/1 -> 1/N/1

== system Encoder_Zynq_V25/IncreEncoder_V25/speed/Average_linear_Reg/moving average of 4 and 8 ==
  omega_Measured : Inport
  E : Inport  Port=2
  Add : Sum  Commented=on  Inputs=++++++++
  Add1 : Sum
  Add2 : Sum
  Add3 : Sum  Commented=on  Inputs=++-
  Add4 : Sum  Inputs=+-
  Add5 : Sum  Inputs=+-
  Bit Shift : hdlsllib/Logic and Bit Operations/Bit Shift  Commented=on  mode=Shift Right Arithmetic  N=3
  Bit Shift1 : hdlsllib/Logic and Bit Operations/Bit Shift  mode=Shift Right Arithmetic  N=3
  Bit Shift2 : hdlsllib/Logic and Bit Operations/Bit Shift  mode=Shift Right Arithmetic  N=2
  Terminator7 : Terminator  Commented=on
  Unit Delay Enabled Synchronous{,1..7} (8 alike) : hdlsllib/Discrete/Unit Delay Enabled Synchronous  InitialCondition=0  SampleTime=-1
      settings: SourceProductBaseCode=SL
  delay : Delay  DelayLength=3
  delay1 : Delay  DelayLength=1
  y(k-1) : hdlsllib/Discrete/Unit Delay Enabled Synchronous  InitialCondition=0  SampleTime=-1
      settings: SourceProductBaseCode=SL
  y(k-1)1 : hdlsllib/Discrete/Unit Delay Enabled Synchronous  InitialCondition=0  SampleTime=-1
      settings: SourceProductBaseCode=SL
  omega_moving_average_N8 : Outport
  omega_moving_average_N4 : Outport  Port=2
  wires:
  E/1 -> delay/1
  Unit Delay Enabled Synchronous1/1 -> Unit Delay Enabled Synchronous2/1, Add/3  "omega_delay2"
  Unit Delay Enabled Synchronous/1 -> Add/2, Unit Delay Enabled Synchronous1/1  "omega_delay1"
  omega_Measured/1 -> delay1/1, Unit Delay Enabled Synchronous/1
  Unit Delay Enabled Synchronous2/1 -> Add/4, Unit Delay Enabled Synchronous3/1  "omega_delay3"
  Unit Delay Enabled Synchronous4/1 -> Add/6, Unit Delay Enabled Synchronous5/1  "omega_delay5"
  Unit Delay Enabled Synchronous5/1 -> Add/7, Unit Delay Enabled Synchronous6/1  "omega_delay6"
  Unit Delay Enabled Synchronous6/1 -> Unit Delay Enabled Synchronous7/1, Add/8  "x(k-7)"
  Add/1 -> Bit Shift/1
  Bit Shift/1 -> Terminator7/1
  delay/1 -> Unit Delay Enabled Synchronous/2, Unit Delay Enabled Synchronous1/2, Unit Delay Enabled Synchronous2/2, Unit Delay Enabled Synchronous4/2, Unit Delay Enabled Synchronous3/2, Unit Delay Enabled Synchronous5/2, Unit Delay Enabled Synchronous7/2, Unit Delay Enabled Synchronous6/2, y(k-1)/2, y(k-1)1/2  "enable_delayed"
  delay1/1 -> Add2/2, Add1/2, Add/1  "x(k)"
  y(k-1)/1 -> Add1/1  "y(k-1)"
  Bit Shift1/1 -> omega_moving_average_N8/1  "omega_mov_avg_alt_N8"
  Unit Delay Enabled Synchronous7/1 -> Add4/2  "x(k-8)"
  Unit Delay Enabled Synchronous3/1 -> Add5/2, Add/5, Unit Delay Enabled Synchronous4/1  "x(k-4)"
  Add5/1 -> y(k-1)1/1, Bit Shift2/1
  Bit Shift2/1 -> omega_moving_average_N4/1  "omega_mov_avg_alt_N4"
  y(k-1)1/1 -> Add2/1  "y(k-1)"
  Add4/1 -> y(k-1)/1, Bit Shift1/1
  Add1/1 -> Add4/1
  Add2/1 -> Add5/1

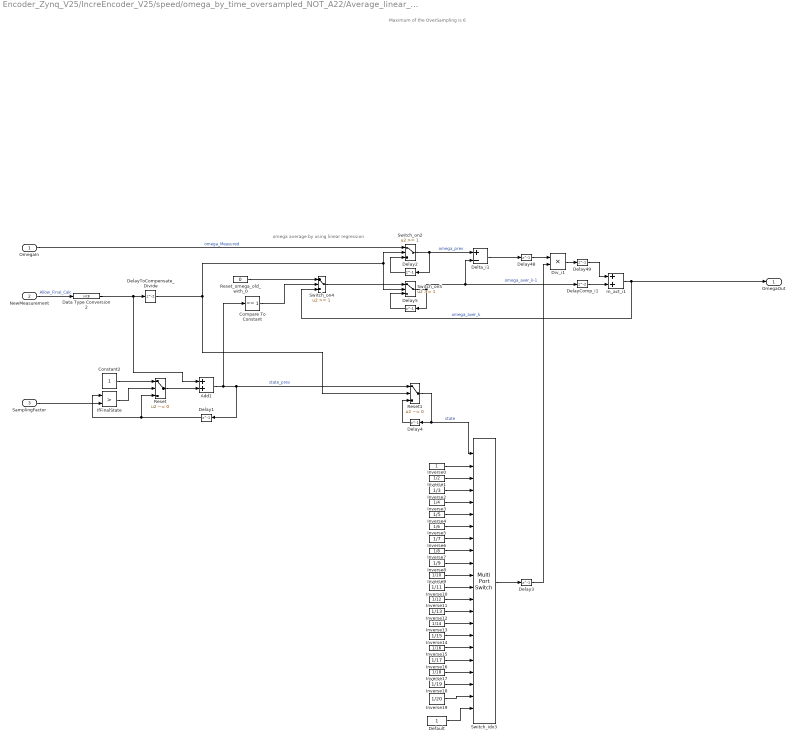
== system Encoder_Zynq_V25/IncreEncoder_V25/speed/omega_by_time_oversampled_NOT_A22/Average_linear_Reg ==
  note: Maximum of the OverSampling is 6
  note: omega average by using linear regression
  "OmegaIn " : Inport
  NewMeasurement : Inport  Port=2
  SamplingFactor : Inport  Port=3
  Add1 : Sum  OutDataTypeStr=Inherit: Same as accumulator
  Compare To Constant : simulink/Logic and Bit Operations/Compare To Constant  relop===  const=1  OutDataTypeStr=boolean
  Constant2 : Constant  OutDataTypeStr=int8  SampleTime=T_50MHz
  Data Type Conversion2 : DataTypeConversion  OutDataTypeStr=int8
  Default : Constant  OutDataTypeStr=fixdt(0,18,18)  SampleTime=-1
  Delay{1..5,48..49} (7 alike) : Delay  DelayLength=1  InitialCondition=0
  DelayComp_i1 : Delay  InitialCondition=0
  DelayToCompensate_Divide : Delay
  Delta_i1 : Sum  Inputs=+-  AccumDataTypeStr=fixdt(1,32,18)  OutDataTypeStr=fixdt(1,24,11)
  Div_i1 : Product  Inputs=**  RndMeth=Simplest  SaturateOnIntegerOverflow=on  OutDataTypeStr=Inherit: Same as first input
  IfFinalState : RelationalOperator  Operator=>  OutDataTypeStr=boolean  RndMeth=Nearest
  Inverse0 : Constant  OutDataTypeStr=fixdt(0,18,18)  SampleTime=-1
  Inverse1 : Constant  Value=1/2  OutDataTypeStr=fixdt(0,18,18)  SampleTime=-1
  Inverse10 : Constant  Value=1/11  OutDataTypeStr=fixdt(0,18,18)  SampleTime=-1
  Inverse11 : Constant  Value=1/12  OutDataTypeStr=fixdt(0,18,18)  SampleTime=-1
  Inverse12 : Constant  Value=1/13  OutDataTypeStr=fixdt(0,18,18)  SampleTime=-1
  Inverse13 : Constant  Value=1/14  OutDataTypeStr=fixdt(0,18,18)  SampleTime=-1
  Inverse14 : Constant  Value=1/15  OutDataTypeStr=fixdt(0,18,18)  SampleTime=-1
  Inverse15 : Constant  Value=1/16  OutDataTypeStr=fixdt(0,18,18)  SampleTime=-1
  Inverse16 : Constant  Value=1/17  OutDataTypeStr=fixdt(0,18,18)  SampleTime=-1
  Inverse17 : Constant  Value=1/18  OutDataTypeStr=fixdt(0,18,18)  SampleTime=-1
  Inverse18 : Constant  Value=1/19  OutDataTypeStr=fixdt(0,18,18)  SampleTime=-1
  Inverse19 : Constant  Value=1/20  OutDataTypeStr=fixdt(0,18,18)  SampleTime=-1
  Inverse2 : Constant  Value=1/3  OutDataTypeStr=fixdt(0,18,18)  SampleTime=-1
  Inverse3 : Constant  Value=1/4  OutDataTypeStr=fixdt(0,18,18)  SampleTime=-1
  Inverse4 : Constant  Value=1/5  OutDataTypeStr=fixdt(0,18,18)  SampleTime=-1
  Inverse5 : Constant  Value=1/6  OutDataTypeStr=fixdt(0,18,18)  SampleTime=-1
  Inverse6 : Constant  Value=1/7  OutDataTypeStr=fixdt(0,18,18)  SampleTime=-1
  Inverse7 : Constant  Value=1/8  OutDataTypeStr=fixdt(0,18,18)  SampleTime=-1
  Inverse8 : Constant  Value=1/9  OutDataTypeStr=fixdt(0,18,18)  SampleTime=-1
  Inverse9 : Constant  Value=1/10  OutDataTypeStr=fixdt(0,18,18)  SampleTime=-1
  Reset : Switch  Criteria=u2 ~= 0  Threshold=0.5  OutDataTypeStr=fixdt(1,24,11)
  Reset1 : Switch  Criteria=u2 ~= 0  Threshold=0.5  OutDataTypeStr=fixdt(1,24,11)
  Reset_omega_old_with_0 : Constant  Value=0  OutDataTypeStr=fixdt(1,24,11)  SampleTime=-1
  Switch_idx3 : MultiPortSwitch  Inputs=20  DataPortForDefault=Additional data port  DiagnosticForDefault=None  OutDataTypeStr=fixdt(0,18,18)  RndMeth=Simplest
  Switch_on2 : Switch  Threshold=1  OutDataTypeStr=fixdt(1,24,11)  RndMeth=Simplest
  Switch_on4 : Switch  Threshold=1  OutDataTypeStr=Inherit: Inherit via back propagation  RndMeth=Simplest
  Switch_on5 : Switch  Threshold=1  OutDataTypeStr=Inherit: Inherit via back propagation  RndMeth=Simplest
  m_act_i1 : Sum  OutDataTypeStr=Inherit: Same as accumulator  RndMeth=Simplest
  OmegaOut : Outport  VectorParamsAs1DForOutWhenUnconnected=off
  wires:
  Delay5/1 -> Switch_on5/3
  NewMeasurement/1 -> Data Type Conversion2/1  "Allow_Final_Calc"
  DelayComp_i1/1 -> m_act_i1/2
  "OmegaIn "/1 -> Switch_on2/1  "omega_Measured"
  m_act_i1/1 -> Switch_on4/3, OmegaOut/1  "omega_aver_k"
  Switch_on5/1 -> DelayComp_i1/1, Delta_i1/2, Delay5/1  "omega_aver_k-1"
  Delay49/1 -> m_act_i1/1
  Delta_i1/1 -> Delay48/1
  Delay48/1 -> Div_i1/1
  Div_i1/1 -> Delay49/1
  Switch_on2/1 -> Delay2/1, Delta_i1/1  "omega_prev"
  Delay2/1 -> Switch_on2/3
  Inverse14/1 -> Switch_idx3/16
  Inverse11/1 -> Switch_idx3/13
  Inverse10/1 -> Switch_idx3/12
  Inverse7/1 -> Switch_idx3/9
  Inverse16/1 -> Switch_idx3/18
  Inverse18/1 -> Switch_idx3/20
  Inverse0/1 -> Switch_idx3/2
  Inverse15/1 -> Switch_idx3/17
  Inverse4/1 -> Switch_idx3/6
  Inverse6/1 -> Switch_idx3/8
  Inverse5/1 -> Switch_idx3/7
  Inverse2/1 -> Switch_idx3/4
  Inverse17/1 -> Switch_idx3/19
  Inverse8/1 -> Switch_idx3/10
  Inverse19/1 -> Switch_idx3/21
  Inverse3/1 -> Switch_idx3/5
  Inverse9/1 -> Switch_idx3/11
  Inverse12/1 -> Switch_idx3/14
  Inverse13/1 -> Switch_idx3/15
  Default/1 -> Switch_idx3/22
  Inverse1/1 -> Switch_idx3/3
  Add1/1 -> Reset1/1, Delay1/1, Compare To Constant/1  "state_prev"
  IfFinalState/1 -> Reset/2
  Reset/1 -> Add1/2
  Constant2/1 -> Reset/1
  Data Type Conversion2/1 -> DelayToCompensate_Divide/1, Add1/1
  Delay1/1 -> Reset/3, IfFinalState/1
  Reset_omega_old_with_0/1 -> Switch_on4/1
  Switch_on4/1 -> Switch_on5/1
  Switch_idx3/1 -> Delay3/1
  Delay3/1 -> Div_i1/2
  Reset1/1 -> Switch_idx3/1, Delay4/1  "state"
  Delay4/1 -> Reset1/3
  DelayToCompensate_Divide/1 -> Switch_on5/2, Switch_on2/2, Reset1/2
  Compare To Constant/1 -> Switch_on4/2
  SamplingFactor/1 -> IfFinalState/2

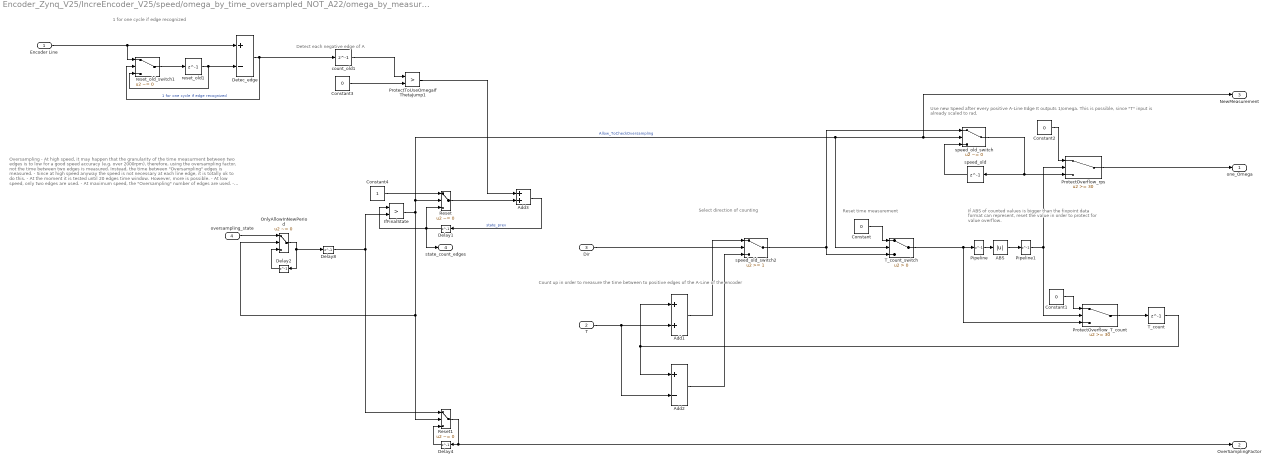
== system Encoder_Zynq_V25/IncreEncoder_V25/speed/omega_by_time_oversampled_NOT_A22/omega_by_measure_time ==
  note: Oversampling
      | - At high speed, it may happen that the granularity of the time measurment between
      | two edges is to low for a good speed accuracy (e.g. over 2000rpm), therefore, using
      | the oversampling factor, not the time between two edges is measured. Instead, the
      | time between "Oversampling" edges is measured.
      | - Since at high speed anyway the speed is not necessary at each line edge,
      |  it is totally ok to do this.
      | - At the moment it is tested until 20 edges time window. However, more is possible.
      | - At low speed, only two edges are used.
      | - At maximum speed, the "Oversampling" number of edges are used.
      | - Between them, a linear factor is used.
      | - Using the OverSampling number also at low speed is not possible,
      |  since the fixpoint range must be quite high! (fixdt(1,36,30) is used at the moment)
  note: Count up in order to measure the time between to positive edges of the A-Line of the encoder
  note: Reset time measurement
  note: 1 for one cycle if edge recognized
  note: Use new Speed after every positive A-Line Edge
      | It outputs 1/omega. This is possible, since "T" input is already scaled to rad.
  note: Select direction of counting
  note: If ABS of counted values is bigger than the
      | fixpoint data format can represent, reset the
      | value in order to protect for value overflow.
  note: Detect each negative edge of A
  Encoder Line : Inport
  T : Inport  Port=2
  Dir : Inport  Port=3
  oversampling_state : Inport  Port=4
  ABS : Abs
  Add1 : Sum  OutDataTypeStr=Inherit: Same as first input
  Add2 : Sum  Inputs=+-  OutDataTypeStr=Inherit: Same as first input
  Add3 : Sum  OutDataTypeStr=Inherit: Same as accumulator
  Constant : Constant  Value=0  OutDataTypeStr=fixdt(1,38,32)  SampleTime=-1
  Constant1 : Constant  Value=0  OutDataTypeStr=fixdt(1,38,32)  SampleTime=-1
  Constant2 : Constant  Value=0  OutDataTypeStr=fixdt(1,38,32)  SampleTime=-1
  Constant3 : Constant  Value=0  OutDataTypeStr=int8  SampleTime=-1
  Constant4 : Constant  OutDataTypeStr=int8  SampleTime=T_50MHz
  Delay{1..2,4,8} (4 alike) : Delay  DelayLength=1  InitialCondition=0
  Detec_edge : Sum  Inputs=+-  AccumDataTypeStr=int8  OutDataTypeStr=int8
  IfFinalState : RelationalOperator  Operator=>  OutDataTypeStr=boolean  RndMeth=Nearest
  OnlyAllowInNewPeriod : Switch  Criteria=u2 ~= 0  Threshold=0.5  OutDataTypeStr=fixdt(0,16,0)
  Pipeline : Delay  DelayLength=1
  Pipeline1 : Delay  DelayLength=1
  ProtectOverflow_T_count : Switch  Threshold=30
  ProtectOverflow_rps : Switch  Threshold=30  OutDataTypeStr=fixdt(1,38,32)
  ProtectToUseOmegaIfThetaJump1 : RelationalOperator  Operator=>  OutDataTypeStr=fixdt(1,16)  RndMeth=Nearest
  Reset : Switch  Criteria=u2 ~= 0  Threshold=0.5  OutDataTypeStr=fixdt(1,24,11)
  Reset1 : Switch  Criteria=u2 ~= 0  Threshold=0.5  OutDataTypeStr=Inherit: Inherit via back propagation
  T_count : Delay  DelayLength=1
  T_count_switch : Switch  Criteria=u2 > Threshold
  count_old1 : Delay  DelayLength=1
  reset_old1 : Delay  DelayLength=1
  reset_old_switch1 : Switch  Criteria=u2 ~= 0
  speed_old : Delay  DelayLength=1
  speed_old_switch : Switch  Criteria=u2 ~= 0  OutDataTypeStr=fixdt(1,38,32)
  speed_old_switch2 : Switch  Threshold=1
  one_Omega : Outport  VectorParamsAs1DForOutWhenUnconnected=off
  OverSamplingFactor : Outport  Port=2  VectorParamsAs1DForOutWhenUnconnected=off
  NewMeasurement : Outport  Port=3  VectorParamsAs1DForOutWhenUnconnected=off
  state_count_edges : Outport  Port=4  VectorParamsAs1DForOutWhenUnconnected=off
  wires:
  Constant/1 -> T_count_switch/1
  Constant1/1 -> ProtectOverflow_T_count/1
  Constant2/1 -> ProtectOverflow_rps/1
  speed_old_switch/1 -> ProtectOverflow_rps/3, speed_old/1
  speed_old/1 -> speed_old_switch/3
  T/1 -> Add1/2, Add2/2
  ProtectOverflow_T_count/1 -> T_count/1
  T_count/1 -> Add2/1, Add1/1
  speed_old_switch2/1 -> speed_old_switch/1, T_count_switch/3
  count_old1/1 -> ProtectToUseOmegaIfThetaJump1/1
  Constant3/1 -> ProtectToUseOmegaIfThetaJump1/2
  Encoder Line/1 -> reset_old_switch1/1, Detec_edge/1
  reset_old_switch1/1 -> reset_old1/1
  reset_old1/1 -> reset_old_switch1/3, Detec_edge/2
  Detec_edge/1 -> reset_old_switch1/2, count_old1/1  "1 for one cycle if edge recognized"
  Dir/1 -> speed_old_switch2/2
  Add1/1 -> speed_old_switch2/1
  Add2/1 -> speed_old_switch2/3
  T_count_switch/1 -> Pipeline/1, ProtectOverflow_T_count/3
  ABS/1 -> Pipeline1/1
  Pipeline/1 -> ABS/1
  Pipeline1/1 -> ProtectOverflow_T_count/2, ProtectOverflow_rps/2
  IfFinalState/1 -> OnlyAllowInNewPeriod/2, Reset1/2, NewMeasurement/1, speed_old_switch/2, T_count_switch/2, Reset/2  "Allow_ToCheckOversampling"
  OnlyAllowInNewPeriod/1 -> Delay8/1, Delay2/1
  Delay1/1 -> state_count_edges/1, Reset/3, IfFinalState/1
  Add3/1 -> Delay1/1  "state_prev"
  Reset/1 -> Add3/2
  Constant4/1 -> Reset/1
  Reset1/1 -> Delay4/1, OverSamplingFactor/1
  Delay2/1 -> OnlyAllowInNewPeriod/3
  ProtectOverflow_rps/1 -> one_Omega/1
  Delay4/1 -> Reset1/3
  Delay8/1 -> Reset1/1, IfFinalState/2
  ProtectToUseOmegaIfThetaJump1/1 -> Add3/1
  oversampling_state/1 -> OnlyAllowInNewPeriod/1
